simulink model "untitled"  (R2022b)
settings: Solver=VariableStepAuto  StartTime=0.0  StopTime=10  RelTol=1e-3
settings Model: Creator=srikar  LastModifiedBy=srikar

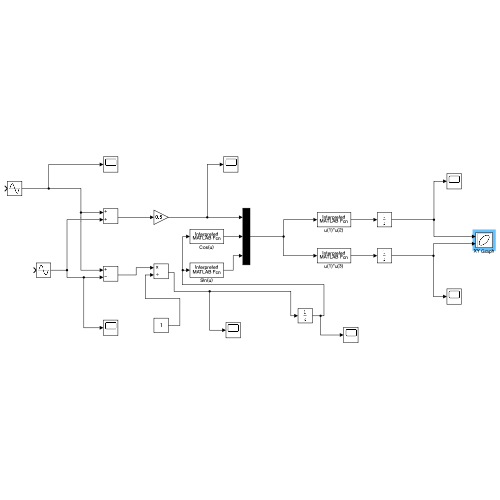
[thumbnail: Simulink's stored preview of the top-level diagram]
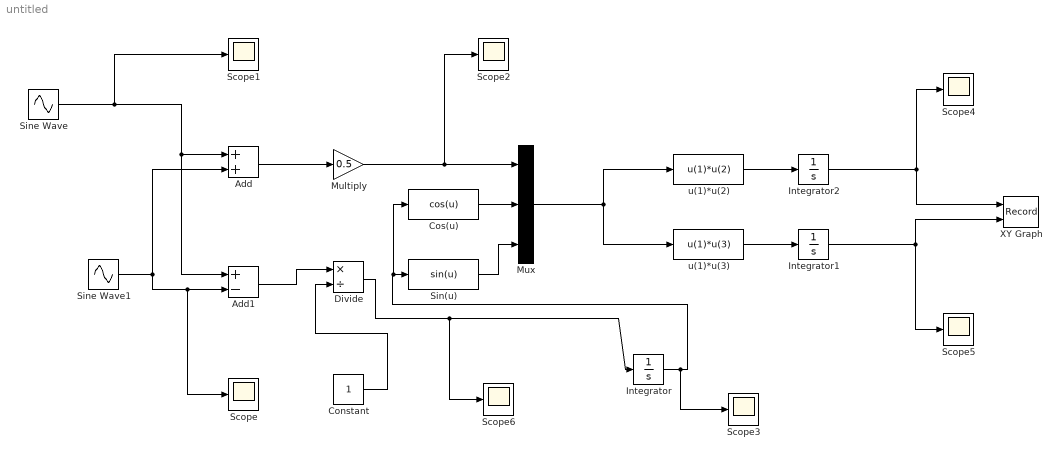
== system untitled ==
  Add : Sum
  Add1 : Sum  Inputs=+-
  Constant : Constant
  Cos(u) : MATLABFcn  MATLABFcn=cos(u)
  Divide : Product  Inputs=*/
  Integrator : Integrator  InitialCondition=pi/2
  Integrator1 : Integrator
  Integrator2 : Integrator
  Multiply : Gain  Gain=0.5
  Mux : Mux  Inputs=3
  Scope{,1..6} (7 alike) : Scope
  Sin(u) : MATLABFcn  MATLABFcn=sin(u)
  Sine Wave : Sin  TimeSource=Use external signal  Bias=1  Phase=pi/4  SampleTime=10
  Sine Wave1 : Sin  TimeSource=Use external signal  Bias=0.5  Frequency=2  Phase=1  SampleTime=10
  XY Graph : Record  FileSettingsInternal="{\"entries\":[{\"content\":{\"excelSettings\":{\"content\":{},\"type\":\"Streamout.ExcelSettings\"}},\"type\":\"Streamout.FileSettingStorage\",\"uuid\":\"478e911c-5aa9-4e8f-9f0d-157409c9e897\"}],\"packageUris\":[\"http://schema.mathworks.com/mf0/streamout_blocks/R2020a\"],\"version\":\"1.0\"}"  Layout=[1 1]  SignalsInternal="{\"entries\":[{\"content\":{\"signals\":[{\"content\":{\"blockPath\":[\"untitled/XY Graph\"],\"channel\":[],\"dimensions\":[1],\"domain\":\"untitled/XY Graph\",\"lineColor\":\"#a2142f\",\"plots\":[1],\"port\":1,\"sid\":[\"\"],\"signalID\":5605,\"signalName\":\"Integrator2\"},\"type\":\"RecordBlkView.Signal\",\"uuid\":\"1fe1e2b7-bdc2-4471-bca0-ed8ebe25cf8f\"},{\"content\":{\"blockPath\":[\"untitled/XY Graph\"],\"channel\":[],\"dimensions\":[1],\"domain\":\"untitled/XY Graph\",\"lineColor\":\"#139fff\",\"plots\":[1],\"port\":2,\"sid\":[\"\"],\"signalID\":5609,\"signalName\":\"Integrator1\"},\"type\":\"RecordBlkView.Signal\",\"uuid\":\"48ee436d-61b3-4c8e-ad8d-f4f53ce4c4ca\"}]},\"type\":\"RecordBlkView.InputSignals\",\"uuid\":\"3ba85647-fbac-4fbe-bd56-6e516d1b5320\"}],\"packageUris\":[\"http://schema.mathworks.com/mf0/streamout_blocks/R2020a\"],\"version\":\"1.0\"}"  VisualizationBindings="{\"xyplotplugin\":{\"info\":[{\"series\":[{\"bindingParametersList\":[{\"parameter\":\"X-Axis\",\"signalID\":5605,\"signalName\":\"Integrator2\"},{\"parameter\":\"Y-Axis\",\"signalID\":5609,\"signalName\":\"Integrator1\"}],\"seriesID\":4745}],\"subplotID\":1}]}}"  CompatibilityTag=XY
  u(1)*u(2) : MATLABFcn  MATLABFcn=u(1)*u(2)
  u(1)*u(3) : MATLABFcn  MATLABFcn=u(1)*u(3)
  wires:
  Add/1 -> Multiply/1
  Sine Wave1/1 -> Scope/1, Add1/2, Add/2
  Add1/1 -> Divide/1
  Constant/1 -> Divide/2
  Mux/1 -> u(1)*u(3)/1, u(1)*u(2)/1
  Multiply/1 -> Scope2/1, Mux/1
  Cos(u)/1 -> Mux/2
  Sin(u)/1 -> Mux/3
  Divide/1 -> Scope6/1, Integrator/1
  Integrator/1 -> Scope3/1, Cos(u)/1, Sin(u)/1
  u(1)*u(2)/1 -> Integrator2/1
  u(1)*u(3)/1 -> Integrator1/1
  Integrator2/1 -> Scope4/1, XY Graph/1
  Integrator1/1 -> Scope5/1, XY Graph/2
  Sine Wave/1 -> Add/1, Add1/1, Scope1/1
